simulink model "imvertpen"  (Simulink 8.7)
settings: Solver=VariableStepAuto  StartTime=0.0  StopTime=10.0  RelTol=1e-3
values from neighbouring files (symbols this model uses):
  g = 9.78    [lab4prelab.m]
  l = 0.303    [lab4prelab.m]
  M = 0.455    [lab4prelab.m]
  m = 0.210    (= 0.21)    [lab4prelab.m]
settings Model: Creator=vukovic8  LastModifiedBy=vukovic8
settings DataIOCC: LimitDataPoints=off  SaveFormat=Dataset
settings DebuggingCC: UnderspecifiedInitializationDetection=Simplified  MergeDetectMultiDrivingBlocksExec=error
settings HardwareCC: ProdBitPerPointer=64  ProdLargestAtomicFloat=Float  ProdIntDivRoundTo=Zero  ProdEndianess=LittleEndian  ProdWordSize=64  ProdHWDeviceType=Intel->x86-64 (Windows64)
settings ModelReferenceCC: PropagateSignalLabelsOutOfModel=on
settings ConfigComp: CovModelRefEnable=off

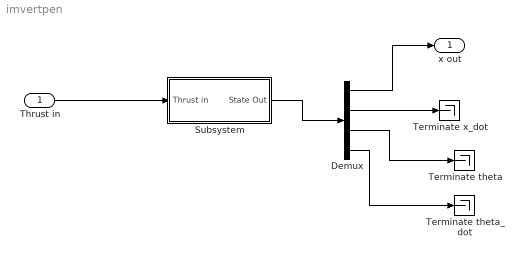
== system imvertpen ==
  Thrust in : Inport
  Demux : Demux
  Subsystem : Subsystem
  Terminate theta : Terminator
  Terminate theta_dot : Terminator
  Terminate x_dot : Terminator
  x out : Outport
  wires:
  Subsystem/1(State Out) -> Demux/1
  Thrust in/1 -> Subsystem/1(Thrust in)
  Demux/1 -> x out/1
  Demux/2 -> Terminate x_dot/1
  Demux/3 -> Terminate theta/1
  Demux/4 -> Terminate theta_dot/1

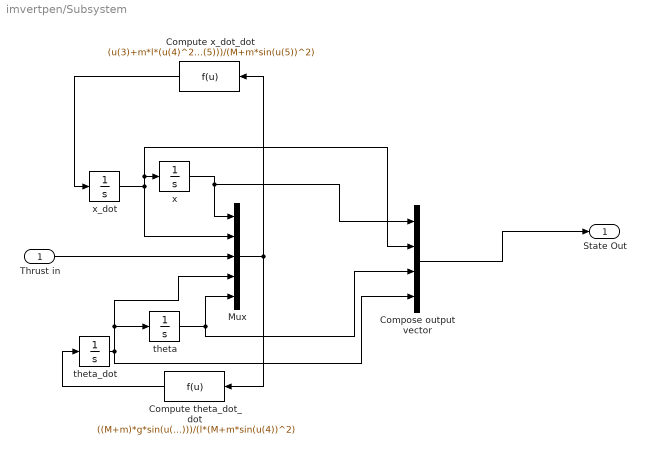
== system imvertpen/Subsystem ==
  Thrust in : Inport
  Compose output vector : Mux
  Compute theta_dot_dot : Fcn  Expr=((M+m)*g*sin(u(5))-u*cos(u(5))-m*l*(u(4))^2*sin(u(5))*cos(u(5)))/(l*(M+m*sin(u(4))^2)
  Compute x_dot_dot : Fcn  Expr=(u(3)+m*l*(u(4)^2)*sin(u(5)) - m*g*cos(u(5))*sin(u(5)))/(M+m*sin(u(5))^2)
  Mux : Mux  Inputs=5
  theta : Integrator
  theta_dot : Integrator
  x : Integrator
  x_dot : Integrator
  State Out : Outport
  wires:
  Thrust in/1 -> Mux/3
  Mux/1 -> Compute x_dot_dot/1, Compute theta_dot_dot/1
  Compute theta_dot_dot/1 -> theta_dot/1
  theta_dot/1 -> theta/1, Mux/4, Compose output vector/4
  theta/1 -> Mux/5, Compose output vector/3
  Compute x_dot_dot/1 -> x_dot/1
  x_dot/1 -> Compose output vector/2, x/1, Mux/2
  x/1 -> Compose output vector/1, Mux/1
  Compose output vector/1 -> State Out/1
